simulink model "electroMagModel"  (R2017b)
settings: Solver=VariableStepAuto  StartTime=0.0  StopTime=5  RelTol=1e-3
undefined symbols (not defined in the file): k1, k2, k3, Ki, Ks, L, m1, m2, m3, R, u_0, x_0
settings Model: Creator=lasse  LastModifiedBy=lasse

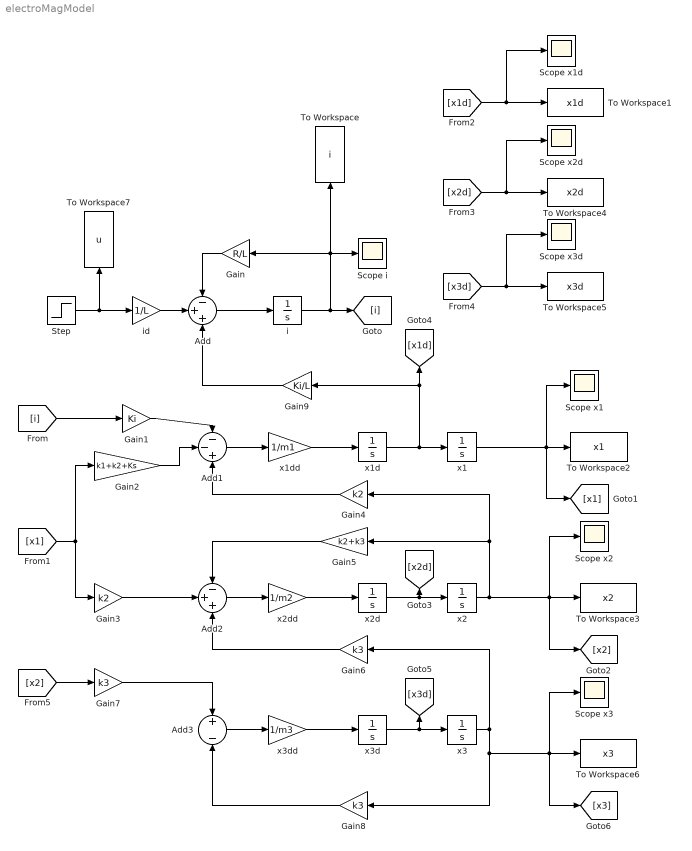
== system electroMagModel ==
  Add : Sum  Inputs=-++
  Add1 : Sum  Inputs=--+
  Add2 : Sum  Inputs=-++
  Add3 : Sum  Inputs=+-
  Gain : Gain  Gain=R/L
  Gain1 : Gain  Gain=Ki
  Gain2 : Gain  Gain=k1+k2+Ks
  Gain3 : Gain  Gain=k2
  Gain4 : Gain  Gain=k2
  Gain5 : Gain  Gain=k2+k3
  Gain6 : Gain  Gain=k3
  Gain7 : Gain  Gain=k3
  Gain8 : Gain  Gain=k3
  Gain9 : Gain  Gain=Ki/L
  Scope i : Scope
  Scope x1 : Scope
  Scope x1d : Scope
  Scope x2 : Scope
  Scope x2d : Scope
  Scope x3 : Scope
  Scope x3d : Scope
  Step : Step  After=u_0  SampleTime=0
  To Workspace : ToWorkspace  VariableName=i  SaveFormat=Structure With Time  SampleTime=-1
  To Workspace1 : ToWorkspace  VariableName=x1d  SaveFormat=Timeseries  SampleTime=-1
  To Workspace2 : ToWorkspace  VariableName=x1  SaveFormat=Timeseries  SampleTime=-1
  To Workspace3 : ToWorkspace  VariableName=x2  SaveFormat=Timeseries  SampleTime=-1
  To Workspace4 : ToWorkspace  VariableName=x2d  SaveFormat=Timeseries  SampleTime=-1
  To Workspace5 : ToWorkspace  VariableName=x3d  SaveFormat=Timeseries  SampleTime=-1
  To Workspace6 : ToWorkspace  VariableName=x3  SaveFormat=Timeseries  SampleTime=-1
  To Workspace7 : ToWorkspace  VariableName=u  SaveFormat=Timeseries  SampleTime=-1
  i : Integrator  InitialCondition=x_0(1)
  "id " : Gain  Gain=1/L
  x1 : Integrator  InitialCondition=x_0(3)
  x1d : Integrator  InitialCondition=x_0(2)
  x1dd : Gain  Gain=1/m1
  x2 : Integrator  InitialCondition=x_0(5)
  x2d : Integrator  InitialCondition=x_0(4)
  x2dd : Gain  Gain=1/m2
  x3 : Integrator  InitialCondition=x_0(7)
  x3d : Integrator  InitialCondition=x_0(6)
  x3dd : Gain  Gain=1/m3
  wires:
  Step/1 -> To Workspace7/1, "id "/1
  Gain/1 -> Add/1
  Add/1 -> i/1
  i/1 -> [i], Scope i/1, Gain/1, To Workspace/1
  [i] -> Gain1/1
  Add1/1 -> x1dd/1
  x1dd/1 -> x1d/1
  x1/1 -> [x1], Scope x1/1, To Workspace2/1
  Gain1/1 -> Add1/1
  Gain2/1 -> Add1/2
  Gain3/1 -> Add2/2
  [x1] -> Gain2/1, Gain3/1
  Add2/1 -> x2dd/1
  x2dd/1 -> x2d/1
  x2d/1 -> [x2d], x2/1
  Gain4/1 -> Add1/3
  Gain5/1 -> Add2/1
  x2/1 -> [x2], Scope x2/1, To Workspace3/1, Gain5/1, Gain4/1
  [x1d] -> Scope x1d/1, To Workspace1/1
  x1d/1 -> Gain9/1, [x1d], x1/1
  [x2d] -> Scope x2d/1, To Workspace4/1
  [x3d] -> Scope x3d/1, To Workspace5/1
  Add3/1 -> x3dd/1
  x3dd/1 -> x3d/1
  Gain6/1 -> Add2/3
  [x2] -> Gain7/1
  Gain7/1 -> Add3/1
  Gain8/1 -> Add3/2
  x3d/1 -> [x3d], x3/1
  x3/1 -> Gain6/1, [x3], Scope x3/1, To Workspace6/1, Gain8/1
  Gain9/1 -> Add/3
  "id "/1 -> Add/2
